simulink library "TransformMatrix"  (R2014b)
settings: Solver=ode45  StartTime=0.0  StopTime=10.0  RelTol=1e-3
settings Model: Creator=Hp  LastModifiedBy=Hp

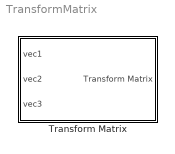
== system TransformMatrix ==
  Transform Matrix : Subsystem

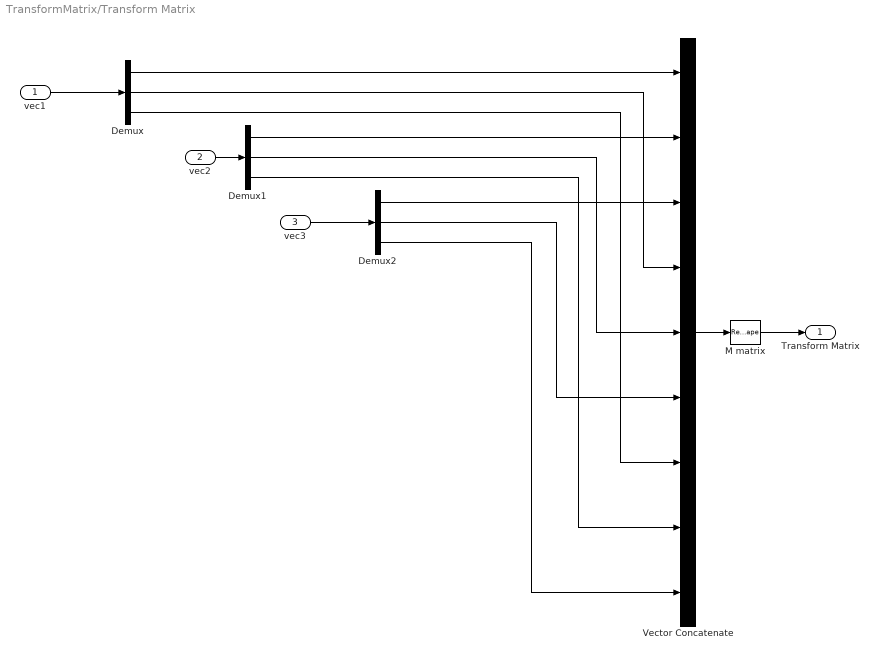
== system TransformMatrix/Transform Matrix ==
  vec1 : Inport
  vec2 : Inport  Port=2
  vec3 : Inport  Port=3
  Demux : Demux  Outputs=3
  Demux1 : Demux  Outputs=3
  Demux2 : Demux  Outputs=3
  M matrix : Reshape  OutputDimensionality=Customize  OutputDimensions=[3,3]
  Vector Concatenate : Concatenate  NumInputs=9
  Transform Matrix : Outport
  wires:
  vec2/1 -> Demux1/1
  vec1/1 -> Demux/1
  Vector Concatenate/1 -> M matrix/1
  Demux1/1 -> Vector Concatenate/2
  Demux/1 -> Vector Concatenate/1
  Demux1/2 -> Vector Concatenate/5
  Demux/3 -> Vector Concatenate/7
  Demux2/3 -> Vector Concatenate/9
  M matrix/1 -> Transform Matrix/1
  Demux/2 -> Vector Concatenate/4
  Demux1/3 -> Vector Concatenate/8
  Demux2/2 -> Vector Concatenate/6
  Demux2/1 -> Vector Concatenate/3
  vec3/1 -> Demux2/1
